simulink model "sampleModel1395_4"  (R2023a)
settings: Solver=VariableStepAuto  StartTime=0.0  StopTime=10.0  RelTol=1e-3
libraries: simulink x1, hdlsllib x1
settings Model: Creator=user1  LastModifiedBy=user1

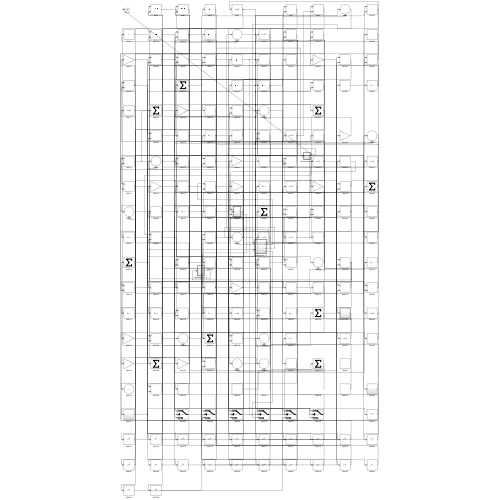
[thumbnail: Simulink's stored preview of the top-level diagram]
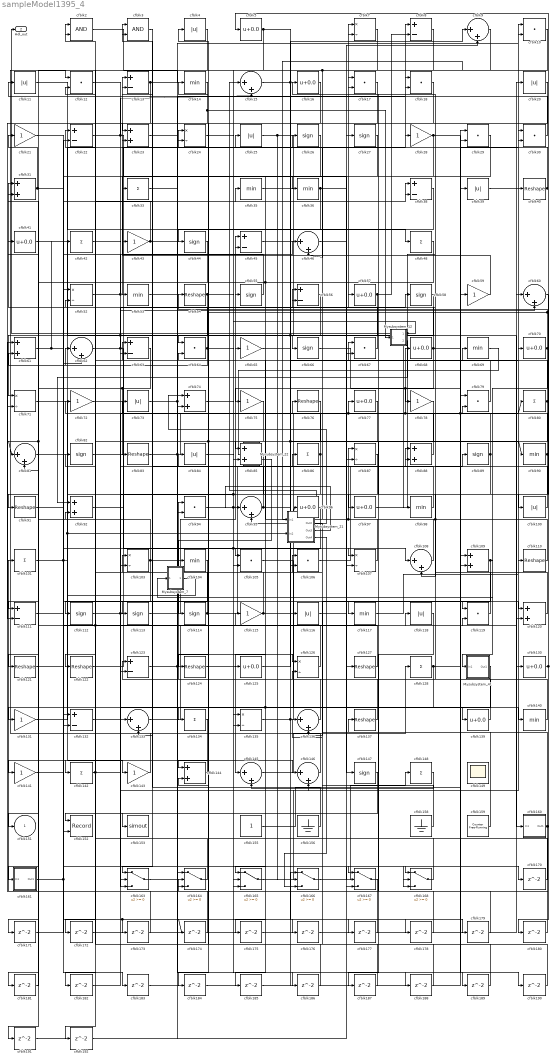
== system sampleModel1395_4 ==
  Mysubsystem_12 : Subsystem  TreatAsAtomicUnit=on  RTWFcnName=Mysubsystem_12
      settings: RTWFcnNameOpts=User specified  RTWFileNameOpts=Use function name
  Mysubsystem_21 : Subsystem  TreatAsAtomicUnit=on  RTWFcnName=Mysubsystem_21
      settings: RTWFcnNameOpts=User specified  RTWFileNameOpts=Use function name
  Mysubsystem_22 : Subsystem  TreatAsAtomicUnit=on  RTWFcnName=Mysubsystem_22
      settings: RTWFcnNameOpts=User specified  RTWFileNameOpts=Use function name
  Mysubsystem_41 : Subsystem  TreatAsAtomicUnit=on  RTWFcnName=Mysubsystem_41
      settings: RTWFcnNameOpts=User specified  RTWFileNameOpts=Use function name
  Mysubsystem_7 : Subsystem  TreatAsAtomicUnit=on  RTWFcnName=Mysubsystem_7
      settings: RTWFcnNameOpts=User specified  RTWFileNameOpts=Use function name
  cfblk{10,12,17..18,29..30,64,67,79,94,105..106,119} (13 alike) : DotProduct  OutDataTypeStr=uint8
  cfblk{4,11,20,25,39,73,84,100,116,118} (10 alike) : Abs  OutDataTypeStr=uint8  SaturateOnIntegerOverflow=off
  cfblk{33,42,48,80,86,101,128,134,142,148} (10 alike) : Sum  Inputs=+  OutDataTypeStr=uint8
  cfblk{7,24,52,71,87,103,107,126,135} (9 alike) : Product  Inputs=*/  OutDataTypeStr=uint8  RndMeth=Zero  SaturateOnIntegerOverflow=on
  cfblk{14,35..36,53,69,90,98,104,117,140} (10 alike) : MinMax  OutDataTypeStr=uint8
  cfblk{9,15,46,60,62,81,95,108,133,136,145..146} (12 alike) : Sum  Inputs=|++  OutDataTypeStr=uint8
  cfblk{23,31,61,74,85,88,92,109,120,144} (10 alike) : Sum  OutDataTypeStr=uint8
  cfblk{40,54,76,83,91,110,121..122,124,127,137} (11 alike) : Reshape
  cfblk{8,13,22,38,45,56,63,111,123,132} (10 alike) : Sum  Inputs=+-  OutDataTypeStr=uint8
  cfblk{26..27,44,55,58,66,82,89,112..114,147} (12 alike) : Signum
  cfblk{21,28,43,59,65,72,75,78,115,131,141,143} (12 alike) : Gain  OutDataTypeStr=uint8
  cfblk{5,16,41,57,68,70,77,96..97,125,130,139} (12 alike) : Bias  Bias=0.0  SaturateOnIntegerOverflow=off
  cfblk149 : Scope
      settings: Floating=on
  cfblk152 : Record  FileSettingsInternal="{\"entries\":[{\"content\":{\"excelSettings\":{\"content\":{},\"type\":\"Streamout.ExcelSettings\"}},\"type\":\"Streamout.FileSettingStorage\",\"uuid\":\"\"}],\"packageUris\":[\"http:\\/\\/schema.mathworks.com\\/mf0\\/streamout_blocks\\/R2020a\"],\"version\":\"1.0\"}"  Layout=[1 1]  SignalsInternal="{\"entries\":[{\"content\":{\"signals\":[{\"content\":{\"blockPath\":[],\"dimensions\":[1],\"domain\":\"\",\"lineColor\":\"#a2142f\",\"plots\":[1],\"port\":1,\"signalID\":10098,\"signalName\":\"cfblk128\"},\"type\":\"RecordBlkView.Signal\",\"uuid\":\"\"},{\"content\":{\"blockPath\":[],\"dimensions\":[1],\"domain\":\"\",\"lineColor\":\"#139fff\",\"plots\":[1],\"port\":2,\"signalID\":10101,\"signalName\":\"cfblk26\"},\"type\":\"RecordBlkView.Signal\",\"uuid\":\"\"}]},\"type\":\"RecordBlkView.InputSignals\",\"uuid\":\"\"}],\"packageUris\":[\"http:\\/\\/schema.mathworks.com\\/mf0\\/streamout_blocks\\/R2020a\"],\"version\":\"1.0\"}"  VisualizationBindings="{\"xyplotplugin\":{\"info\":[{\"series\":[{\"bindingParametersList\":[{\"parameter\":\"X-Axis\",\"signalID\":10098,\"signalName\":\"cfblk128\"},{\"parameter\":\"Y-Axis\",\"signalID\":10101,\"signalName\":\"cfblk26\"}],\"seriesID\":10540}],\"subplotID\":1}]}}"  CompatibilityTag=XY  st=-1
  cfblk153 : ToWorkspace  VariableName=simout  SaveFormat=Timeseries  SampleTime=-1
  cfblk155 : Constant  OutDataTypeStr=uint8  SampleTime=-1
  cfblk156 : Ground
  cfblk158 : Ground
  cfblk159 : hdlsllib/Sources/Counter Free-Running  NumBits=16  tsamp=-1
  cfblk160 : Subsystem
      settings: LibrarySourceBlock=|
      | hdlsllib/Ports &
      | Subsystems/Subsystem
  cfblk161 : Subsystem
      settings: LibrarySourceBlock=|
      | hdlsllib/Ports &
      | Subsystems/Subsystem
  cfblk{163..168} (6 alike) : Switch  OutDataTypeStr=uint8  SaturateOnIntegerOverflow=off  InputSameDT=off
  cfblk{170..192} (23 alike) : Delay  SampleTime=1
  cfblk2 : Logic  AllPortsSameDT=off  OutDataTypeStr=boolean
  cfblk3 : Logic  AllPortsSameDT=off  OutDataTypeStr=boolean
  cfblk151 : Outport  OutDataTypeStr=uint8  VectorParamsAs1DForOutWhenUnconnected=off
  Hdl_out : Outport  Port=2  OutDataTypeStr=uint8
  wires:
  cfblk92/1 -> cfblk108/1
  cfblk165/1 -> cfblk10/1
  cfblk11/1 -> cfblk48/1
  cfblk112/1 -> cfblk117/1, cfblk88/2
  cfblk97/1 -> cfblk16/1
  cfblk143/1 -> cfblk12/1
  cfblk79/1 -> cfblk22/1
  cfblk122/1 -> cfblk58/1
  cfblk131/1 -> cfblk8/1
  cfblk36/1 -> cfblk9/2, cfblk175/1
  cfblk136/1 -> cfblk94/1
  cfblk70/1 -> Mysubsystem_41/1(In1), cfblk54/1, cfblk4/1
  cfblk114/1 -> cfblk88/1, cfblk82/1
  cfblk72/1 -> cfblk25/1
  cfblk15/1 -> cfblk90/1, cfblk168/3, cfblk67/2, cfblk7/2
  cfblk28/1 -> cfblk53/1, cfblk190/1
  cfblk113/1 -> cfblk45/1
  cfblk160/1(Out1) -> cfblk101/1, cfblk95/2
  cfblk41/1 -> cfblk160/1(In1)
  cfblk101/1 -> cfblk143/1, cfblk45/2
  cfblk106/1 -> cfblk89/1
  cfblk9/1 -> cfblk112/1
  cfblk108/1 -> cfblk87/1, cfblk73/1
  cfblk46/1 -> cfblk87/2
  cfblk64/1 -> cfblk13/1, cfblk61/2, cfblk167/2
  cfblk145/1 -> cfblk128/1
  cfblk121/1 -> cfblk62/2
  cfblk8/1 -> cfblk111/1
  cfblk83/1 -> cfblk76/1, cfblk38/1
  cfblk105/1 -> cfblk140/1
  cfblk159/1 -> cfblk103/1
  cfblk124/1 -> cfblk145/1
  cfblk2/1 -> cfblk74/2
  cfblk62/1 -> cfblk114/1, cfblk57/1
  cfblk57/1 -> cfblk131/1, cfblk163/3, cfblk8/2
  cfblk123/1 -> cfblk118/1, cfblk188/1
  cfblk135/1 -> cfblk59/1, cfblk179/1
  cfblk55/1 -> cfblk13/2
  cfblk73/1 -> cfblk18/2, cfblk189/1
  cfblk24/1 -> cfblk66/1
  cfblk100/1 -> cfblk28/1
  cfblk146/1 -> cfblk12/2
  cfblk89/1 -> cfblk68/1, cfblk2/2, cfblk105/2
  cfblk12/1 -> cfblk139/1
  cfblk71/1 -> cfblk147/1
  cfblk35/1 -> cfblk98/1
  cfblk95/1 -> cfblk84/1, cfblk38/2
  cfblk52/1 -> cfblk64/1, cfblk46/1
  cfblk68/1 -> cfblk78/1, cfblk105/1, cfblk31/1, cfblk120/2
  cfblk67/1 -> cfblk7/1
  cfblk156/1 -> cfblk63/1
  cfblk75/1 -> cfblk142/1
  cfblk109/1 -> Mysubsystem_7/1(In1), cfblk136/2
  cfblk31/1 -> cfblk21/1, cfblk120/1
  cfblk119/1 -> cfblk96/1, cfblk56/2
  cfblk7/1 -> cfblk153/1, cfblk46/2
  cfblk86/1 -> cfblk113/1, cfblk23/2
  cfblk4/1 -> cfblk122/1
  cfblk18/1 -> cfblk63/2
  cfblk77/1 -> cfblk85/1
  cfblk90/1 -> cfblk77/1, cfblk65/1, cfblk108/2
  cfblk80/1 -> cfblk69/1, cfblk97/1
  cfblk17/1 -> cfblk44/1
  cfblk44/1 -> cfblk161/1(In1)
  cfblk120/1 -> cfblk67/1
  cfblk48/1 -> cfblk165/1, cfblk181/1
  cfblk142/1 -> cfblk146/2, cfblk192/1
  cfblk115/1 -> cfblk14/1, cfblk9/1
  cfblk59/1 -> cfblk43/1
  cfblk144/1 -> cfblk141/1
  cfblk58/1 -> cfblk71/1
  cfblk161/1(Out1) -> cfblk167/1, cfblk176/1
  cfblk29/1 -> cfblk125/1
  cfblk133/1 -> cfblk20/1
  cfblk22/1 -> cfblk107/2, cfblk15/2, cfblk170/1
  cfblk43/1 -> cfblk2/1, cfblk178/1
  cfblk155/1 -> cfblk39/1
  cfblk16/1 -> cfblk111/2
  cfblk13/1 -> cfblk10/2, cfblk71/2
  cfblk78/1 -> cfblk124/1, cfblk163/2
  cfblk163/1 -> cfblk55/1
  cfblk63/1 -> cfblk91/1, cfblk83/1
  cfblk76/1 -> cfblk163/1
  cfblk39/1 -> cfblk40/1
  cfblk85/1 -> cfblk134/1
  cfblk81/1 -> cfblk135/1
  cfblk3/1 -> cfblk23/1
  cfblk65/1 -> cfblk168/1
  cfblk53/1 -> cfblk126/1
  cfblk66/1 -> cfblk109/1
  cfblk98/1 -> cfblk3/1
  cfblk54/1 -> cfblk133/2, cfblk168/2
  cfblk14/1 -> Mysubsystem_12/1(In1), cfblk151/1, cfblk81/1
  cfblk158/1 -> cfblk115/1
  cfblk61/1 -> cfblk173/1, cfblk174/1, cfblk42/1
  cfblk94/1 -> cfblk29/2, cfblk106/2
  cfblk148/1 -> cfblk145/2
  cfblk5/1 -> cfblk116/1, cfblk165/2
  cfblk164/1 -> cfblk92/2
  cfblk166/1 -> cfblk148/1
  cfblk23/1 -> cfblk146/1
  cfblk132/1 -> cfblk79/2
  cfblk82/1 -> cfblk107/1
  cfblk25/1 -> cfblk130/1, cfblk166/2
  cfblk128/1 -> cfblk152/1, cfblk185/1, cfblk30/1, cfblk80/1
  cfblk125/1 -> cfblk70/1
  cfblk42/1 -> cfblk60/2
  cfblk27/1 -> cfblk75/1
  cfblk40/1 -> cfblk5/1, cfblk3/2
  cfblk60/1 -> cfblk100/1
  cfblk26/1 -> cfblk152/2
  cfblk168/1 -> cfblk137/1
  cfblk117/1 -> cfblk110/1
  cfblk139/1 -> cfblk18/1
  cfblk111/1 -> cfblk35/1
  cfblk30/1 -> cfblk11/1
  cfblk140/1 -> cfblk123/1
  cfblk127/1 -> cfblk72/1, cfblk81/2
  cfblk45/1 -> cfblk127/1
  cfblk21/1 -> cfblk52/1
  cfblk167/1 -> cfblk164/2
  cfblk137/1 -> cfblk106/1
  cfblk116/1 -> cfblk119/1
  cfblk88/1 -> cfblk17/1
  cfblk126/1 -> cfblk33/1
  cfblk130/1 -> cfblk30/2, cfblk180/1
  cfblk56/1 -> cfblk121/1
  cfblk87/1 -> cfblk135/2, cfblk103/2
  cfblk20/1 -> cfblk144/1
  cfblk110/1 -> cfblk56/1
  cfblk33/1 -> cfblk36/1
  cfblk107/1 -> cfblk26/1
  cfblk96/1 -> cfblk132/2, cfblk165/3
  cfblk103/1 -> cfblk86/1, cfblk41/1, cfblk123/2
  cfblk141/1 -> cfblk119/2
  cfblk170/1 -> cfblk24/2
  cfblk134/1 -> cfblk171/1
  cfblk171/1 -> cfblk22/2
  cfblk147/1 -> cfblk172/1
  cfblk172/1 -> cfblk29/1
  cfblk173/1 -> cfblk132/1
  cfblk174/1 -> cfblk52/2
  cfblk175/1 -> cfblk79/1
  cfblk176/1 -> cfblk60/1
  cfblk74/1 -> cfblk177/1
  cfblk177/1 -> cfblk126/2
  cfblk178/1 -> cfblk17/2
  cfblk179/1 -> cfblk61/1
  cfblk180/1 -> cfblk164/3
  cfblk181/1 -> cfblk31/2
  cfblk104/1 -> cfblk182/1
  cfblk182/1 -> cfblk133/1
  cfblk91/1 -> cfblk183/1
  cfblk183/1 -> cfblk166/1
  cfblk38/1 -> cfblk184/1
  cfblk184/1 -> cfblk109/2
  cfblk185/1 -> cfblk167/3
  cfblk84/1 -> cfblk186/1
  cfblk186/1 -> cfblk64/2
  cfblk118/1 -> cfblk187/1
  cfblk187/1 -> cfblk62/1
  cfblk188/1 -> cfblk144/2
  cfblk189/1 -> cfblk164/1
  cfblk190/1 -> cfblk136/1
  cfblk191/1 -> cfblk94/2
  cfblk192/1 -> cfblk27/1
  Mysubsystem_7/1(Out1) -> cfblk24/1, Mysubsystem_21/2(In2)
  Mysubsystem_12/1(Out1) -> cfblk85/2, Hdl_out/1
  Mysubsystem_12/2(Out2) -> cfblk92/1
  cfblk10/1 -> Mysubsystem_21/1(In1)
  Mysubsystem_21/1(Out1) -> cfblk15/1
  Mysubsystem_21/2(Out2) -> cfblk74/1
  Mysubsystem_21/3(Out3) -> cfblk95/1
  Mysubsystem_21/4(Out4) -> cfblk166/3
  cfblk69/1 -> Mysubsystem_22/1(In1)
  Mysubsystem_22/1(Out1) -> cfblk104/1
  Mysubsystem_41/1(Out1) -> cfblk191/1

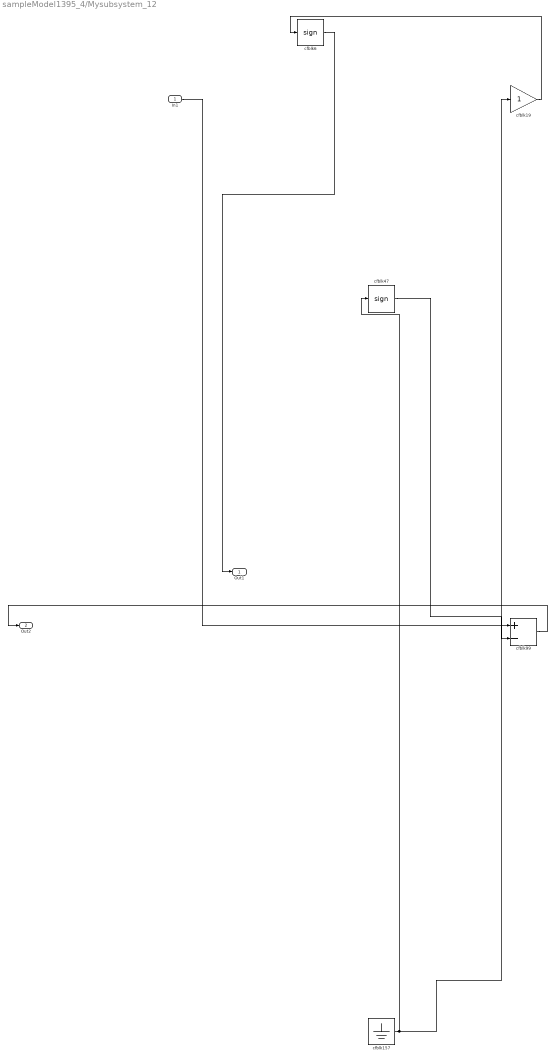
== system sampleModel1395_4/Mysubsystem_12 ==
  In1 : Inport
  cfblk157 : Ground
  cfblk19 : Gain
  cfblk47 : Signum
  cfblk6 : Signum
  cfblk99 : Sum  Inputs=+-
  Out1 : Outport
  Out2 : Outport  Port=2
  wires:
  cfblk157/1 -> cfblk19/1, cfblk47/1
  cfblk19/1 -> cfblk6/1
  cfblk6/1 -> Out1/1
  cfblk99/1 -> Out2/1
  cfblk47/1 -> cfblk99/2
  In1/1 -> cfblk99/1

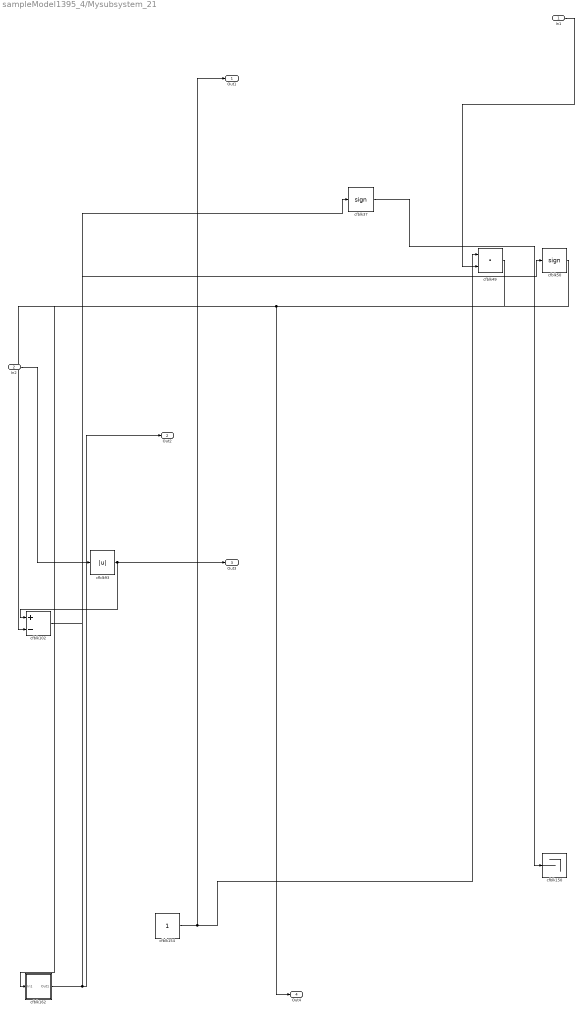
== system sampleModel1395_4/Mysubsystem_21 ==
  In1 : Inport
  In2 : Inport  Port=2
  cfblk102 : Sum  Inputs=+-
  cfblk150 : Terminator
  cfblk154 : Constant  SampleTime=-1
  cfblk162 : Subsystem
      settings: LibrarySourceBlock=|
      | hdlsllib/Ports &
      | Subsystems/Subsystem
  cfblk37 : Signum
  cfblk49 : DotProduct  OutDataTypeStr=Inherit: Inherit via internal rule
  cfblk50 : Signum
  cfblk93 : Abs  SaturateOnIntegerOverflow=off
  Out1 : Outport
  Out2 : Outport  Port=2
  Out3 : Outport  Port=3
  Out4 : Outport  Port=4
  wires:
  In2/1 -> cfblk93/1
  cfblk154/1 -> Out1/1, cfblk49/1
  cfblk102/1 -> cfblk37/1
  cfblk37/1 -> cfblk150/1
  cfblk93/1 -> Out3/1, cfblk162/1(In1)
  cfblk50/1 -> Out4/1, cfblk102/1
  cfblk162/1(Out1) -> Out2/1, cfblk50/1
  cfblk49/1 -> cfblk102/2
  In1/1 -> cfblk49/2

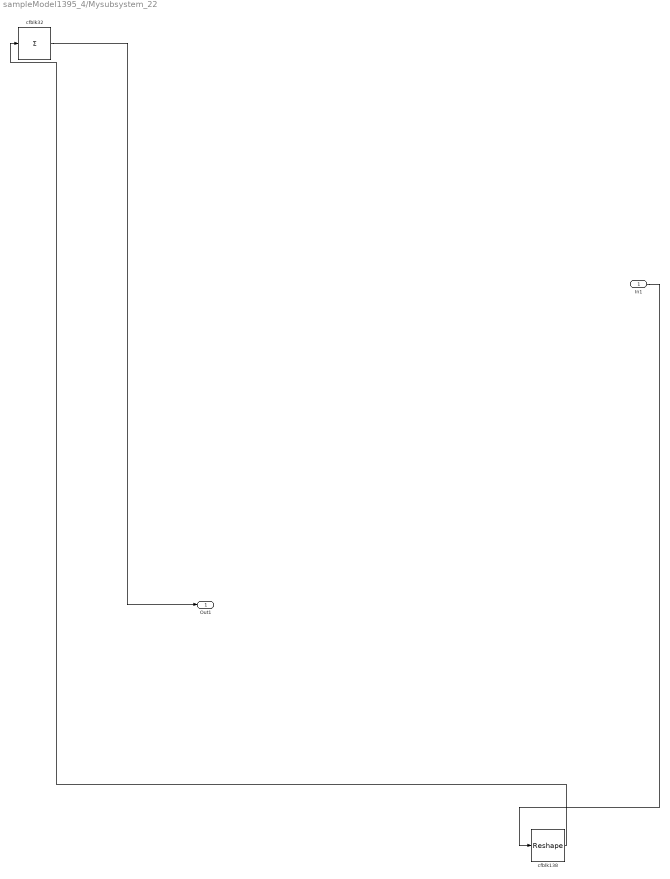
== system sampleModel1395_4/Mysubsystem_22 ==
  In1 : Inport
  cfblk138 : Reshape
  cfblk32 : Sum  Inputs=+
  Out1 : Outport
  wires:
  cfblk138/1 -> cfblk32/1
  In1/1 -> cfblk138/1
  cfblk32/1 -> Out1/1

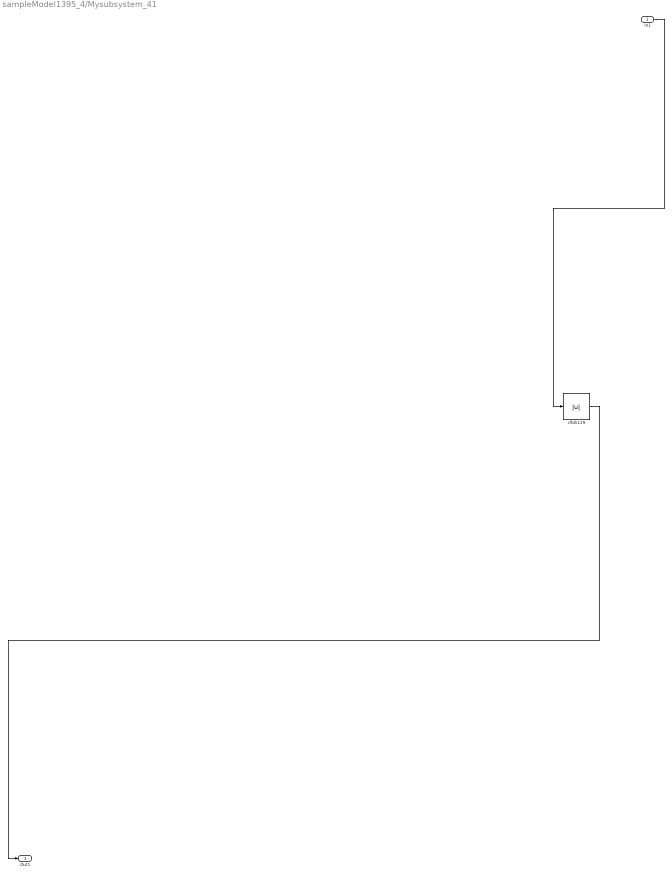
== system sampleModel1395_4/Mysubsystem_41 ==
  In1 : Inport
  cfblk129 : Abs  SaturateOnIntegerOverflow=off
  Out1 : Outport
  wires:
  In1/1 -> cfblk129/1
  cfblk129/1 -> Out1/1

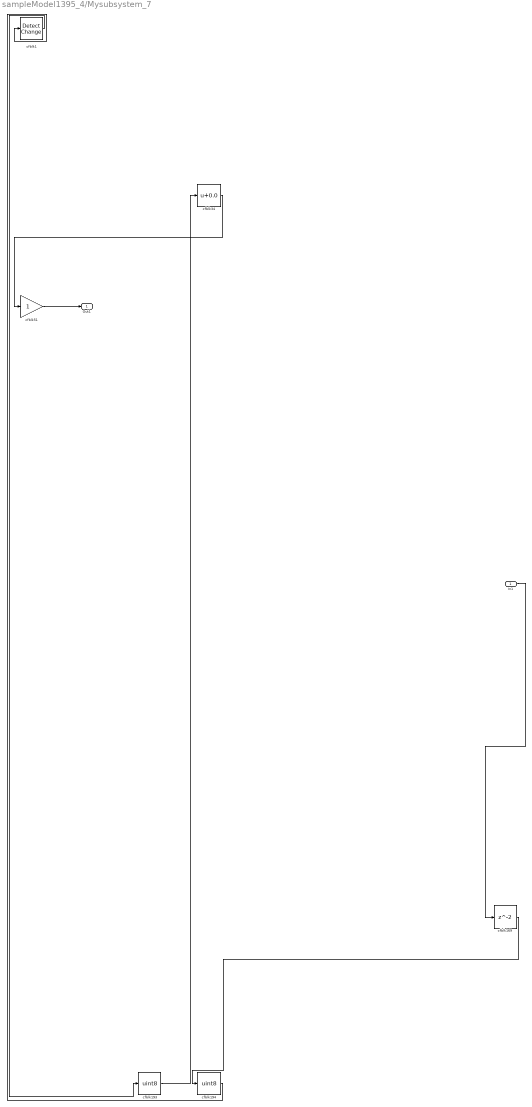
== system sampleModel1395_4/Mysubsystem_7 ==
  In1 : Inport
  cfblk1 : simulink/Logic and Bit Operations/Detect Change  vinit=0  OutDataTypeStr=boolean
      settings: LibrarySourceBlock=|
      | hdlsllib/Logic and Bit
      | Operations/Detect
      | Change
  cfblk169 : Delay  SampleTime=1
  cfblk193 : DataTypeConversion  OutDataTypeStr=uint8  SaturateOnIntegerOverflow=off  RndMeth=Floor
  cfblk194 : DataTypeConversion  OutDataTypeStr=uint8  SaturateOnIntegerOverflow=off  RndMeth=Floor
  cfblk34 : Bias  Bias=0.0  SaturateOnIntegerOverflow=off
  cfblk51 : Gain
  Out1 : Outport
  wires:
  cfblk194/1 -> cfblk1/1
  cfblk1/1 -> cfblk193/1
  cfblk34/1 -> cfblk51/1
  cfblk193/1 -> cfblk34/1
  cfblk169/1 -> cfblk194/1
  In1/1 -> cfblk169/1
  cfblk51/1 -> Out1/1

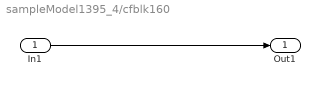
== system sampleModel1395_4/cfblk160 ==
  In1 : Inport
  Out1 : Outport
  wires:
  In1/1 -> Out1/1

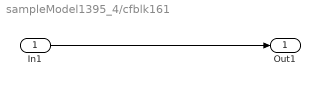
== system sampleModel1395_4/cfblk161 ==
  In1 : Inport
  Out1 : Outport
  wires:
  In1/1 -> Out1/1

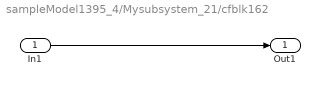
== system sampleModel1395_4/Mysubsystem_21/cfblk162 ==
  In1 : Inport
  Out1 : Outport
  wires:
  In1/1 -> Out1/1
